simulink model "task2"  (R2022b)
settings: Solver=VariableStepAuto  StartTime=0.0  StopTime=10.0  RelTol=1e-3
values from neighbouring files (symbols this model uses):
  I = [0.07, 0.0504, 0.0109]    [task1main.m]    (also in task2main.m = diag(I); task3main.m = diag(I); task4main.m = diag(I); task5.m = [0.07; 0.0109; 0.0504])
  I_inv = pinv(I)    [task2main.m]    (also in task3main.m; task4main.m; task6main.m)
  w0 = [0.45, 0.52, 0.55]    [task1main.m]    (also in task2main.m = [0.45; 0.52; 0.55]; task3main.m = [0.45; 0.52; 0.55]; task4main.m = cat(1,w0,wr0); task5.m = [0.01; 0.01; 2])
libraries: matrix_library x1
settings Model: Creator=a1pab  LastModifiedBy=a1pab

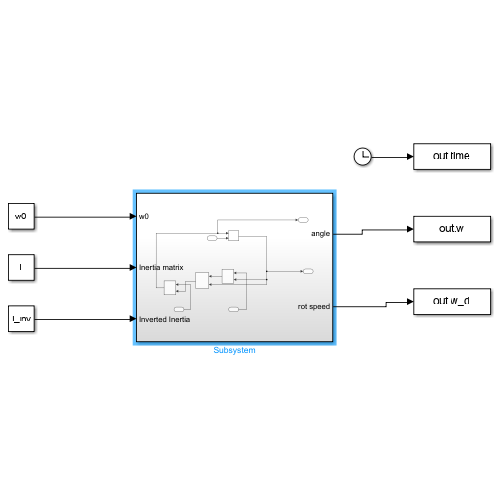
[thumbnail: Simulink's stored preview of the top-level diagram]
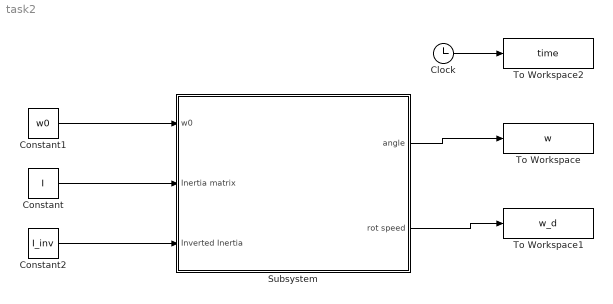
== system task2 ==
  Clock : Clock
  Constant : Constant  Value=I  VectorParams1D=off
  Constant1 : Constant  Value=w0  VectorParams1D=off
  Constant2 : Constant  Value=I_inv  VectorParams1D=off
  Subsystem : Subsystem
  To Workspace : ToWorkspace  VariableName=w  SampleTime=-1
  To Workspace1 : ToWorkspace  VariableName=w_d  SampleTime=-1
  To Workspace2 : ToWorkspace  VariableName=time  SampleTime=-1
  wires:
  Subsystem/1(angle) -> To Workspace/1
  Subsystem/2(rot speed) -> To Workspace1/1
  Constant/1 -> Subsystem/2(Inertia matrix)
  Constant1/1 -> Subsystem/1(w0)
  Clock/1 -> To Workspace2/1
  Constant2/1 -> Subsystem/3(Inverted Inertia)

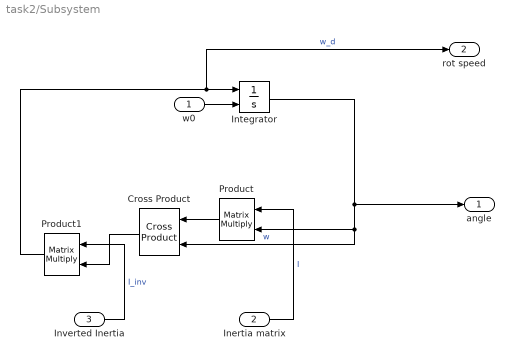
== system task2/Subsystem ==
  w0 : Inport
  Inertia matrix : Inport  Port=2
  Inverted Inertia : Inport  Port=3
  Cross Product : matrix_library/Cross Product
  Integrator : Integrator  InitialConditionSource=external
  Product : Product  Multiplication=Matrix(*)
  Product1 : Product  Multiplication=Matrix(*)
  angle : Outport
  rot speed : Outport  Port=2
  wires:
  Product1/1 -> rot speed/1, Integrator/1  "w_d"
  Integrator/1 -> Cross Product/2, Product/2, angle/1  "w"
  w0/1 -> Integrator/2
  Product/1 -> Cross Product/1
  Cross Product/1 -> Product1/2
  Inverted Inertia/1 -> Product1/1  "I_inv"
  Inertia matrix/1 -> Product/1  "I"
